simulink model "Batbot_SIM"  (Simulink 7.5)
settings: Solver=ode45  StartTime=0.0  StopTime=5  FixedStep=0.1  RelTol=1e-3
values from neighbouring files (symbols this model uses):
  F_flapping = 1000    [SimulationFB.m]
  step_2 = tf/(col-1)    [SimulationFB.m]    (also in inverse_kinematicsFULLFB.m = 0.0114285714286)
libraries: mblibv1 x76, motdrv_lib x8, simulink x7
(part 3 of 3)

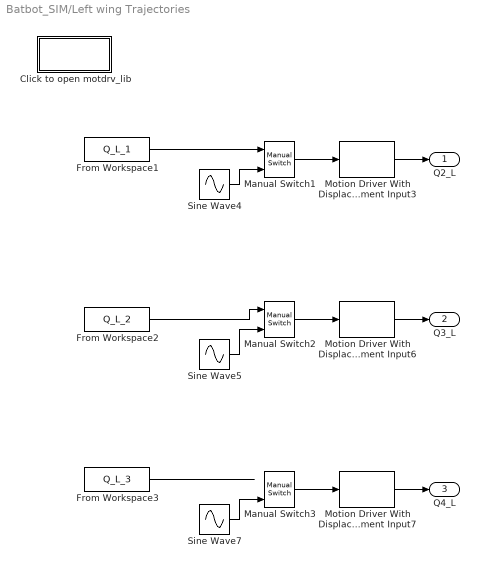
== system Batbot_SIM/Left wing Trajectories  ==
  Click to open motdrv_lib : Subsystem
      settings: OpenFcn=open_system('motdrv_lib');
      mask Type: Double-click to open motdrv_lib
      mask Display: disp('motdrv_lib');
  From Workspace1 : FromWorkspace  VariableName=Q_L_1  SampleTime=step_2  OutputAfterFinalValue=Setting to zero
  From Workspace2 : FromWorkspace  VariableName=Q_L_2  SampleTime=step_2  OutputAfterFinalValue=Setting to zero
  From Workspace3 : FromWorkspace  VariableName=Q_L_3  SampleTime=step_2  OutputAfterFinalValue=Setting to zero
  Manual Switch1 : simulink/Signal Routing/Manual Switch  SystemSampleTime=-1  sw=0  action=0  varsize=off
  Manual Switch2 : simulink/Signal Routing/Manual Switch  SystemSampleTime=-1  sw=0  action=0  varsize=off
  Manual Switch3 : simulink/Signal Routing/Manual Switch  SystemSampleTime=-1  sw=0  action=0  varsize=off
  Motion Driver With Displacement Input3 : motdrv_lib/Motion Driver With Displacement Input  SystemSampleTime=-1  InitialDisplacementSource=Dialog  InitialDisplacement=0  InitialVelocity=0  TimeConstant=1e-3
  Motion Driver With Displacement Input6 : motdrv_lib/Motion Driver With Displacement Input  SystemSampleTime=-1  InitialDisplacementSource=Dialog  InitialDisplacement=0  InitialVelocity=0  TimeConstant=1e-3
  Motion Driver With Displacement Input7 : motdrv_lib/Motion Driver With Displacement Input  SystemSampleTime=-1  InitialDisplacementSource=Dialog  InitialDisplacement=0  InitialVelocity=0  TimeConstant=1e-3
  Sine Wave4 : Sin  Amplitude=40  Bias=0  Frequency=1000  Phase=0  Samples=10  SampleTime=0  Offset=0
  Sine Wave5 : Sin  Amplitude=-60  Bias=0  Frequency=1000  Phase=0  Samples=10  SampleTime=0  Offset=0
  Sine Wave7 : Sin  Amplitude=-60  Bias=0  Frequency=1000  Phase=0  Samples=10  SampleTime=0  Offset=0
  Q2_L : Outport  OutDataType=fixdt(1, 16)  OutScaling=2^0
  Q3_L : Outport  Port=2  OutDataType=fixdt(1, 16)  OutScaling=2^0
  Q4_L : Outport  Port=3  OutDataType=fixdt(1, 16)  OutScaling=2^0
  wires:
  Motion Driver With Displacement Input3/1 -> Q2_L/1
  Motion Driver With Displacement Input6/1 -> Q3_L/1
  Motion Driver With Displacement Input7/1 -> Q4_L/1
  Manual Switch3/1 -> Motion Driver With Displacement Input7/1
  Sine Wave7/1 -> Manual Switch3/2
  Sine Wave5/1 -> Manual Switch2/2
  Sine Wave4/1 -> Manual Switch1/2
  Manual Switch1/1 -> Motion Driver With Displacement Input3/1
  Manual Switch2/1 -> Motion Driver With Displacement Input6/1
  From Workspace1/1 -> Manual Switch1/1
  From Workspace2/1 -> Manual Switch2/1
  From Workspace3/1 -> ?

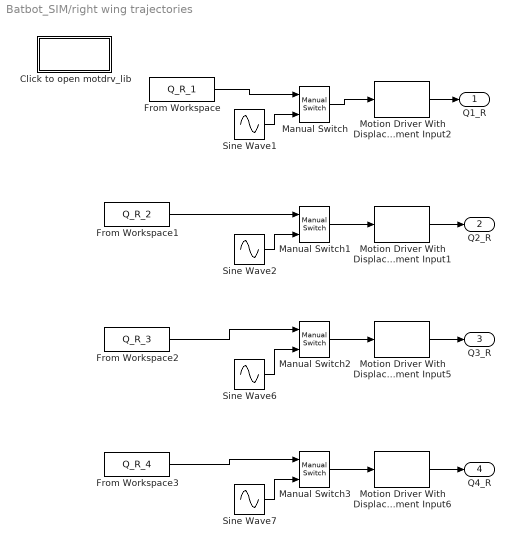
== system Batbot_SIM/right wing trajectories ==
  Click to open motdrv_lib : Subsystem
      settings: OpenFcn=open_system('motdrv_lib');
      mask Type: Double-click to open motdrv_lib
      mask Display: disp('motdrv_lib');
  From Workspace : FromWorkspace  VariableName=Q_R_1  SampleTime=step_2  OutputAfterFinalValue=Setting to zero
  From Workspace1 : FromWorkspace  VariableName=Q_R_2  SampleTime=step_2  OutputAfterFinalValue=Setting to zero
  From Workspace2 : FromWorkspace  VariableName=Q_R_3  SampleTime=step_2  OutputAfterFinalValue=Setting to zero
  From Workspace3 : FromWorkspace  VariableName=Q_R_4  SampleTime=step_2  OutputAfterFinalValue=Setting to zero
  Manual Switch{,1..3} (4 alike) : simulink/Signal Routing/Manual Switch  SystemSampleTime=-1  sw=0  action=0  varsize=off
  Motion Driver With Displacement Input{1..2,5..6} (4 alike) : motdrv_lib/Motion Driver With Displacement Input  SystemSampleTime=-1  InitialDisplacementSource=Dialog  InitialDisplacement=0  InitialVelocity=0  TimeConstant=1e-3
  Sine Wave1 : Sin  Amplitude=200  Bias=0  Frequency=F_flapping  Phase=0  Samples=10  SampleTime=0  Offset=0
  Sine Wave2 : Sin  Amplitude=40  Bias=0  Frequency=1000  Phase=0  Samples=10  SampleTime=0  Offset=0
  Sine Wave6 : Sin  Amplitude=60  Bias=0  Frequency=1000  Phase=0  Samples=10  SampleTime=0  Offset=0
  Sine Wave7 : Sin  Amplitude=60  Bias=0  Frequency=1000  Phase=0  Samples=10  SampleTime=0  Offset=0
  Q1_R : Outport  OutDataType=fixdt(1, 16)  OutScaling=2^0
  Q2_R : Outport  Port=2  OutDataType=fixdt(1, 16)  OutScaling=2^0
  Q3_R : Outport  Port=3  OutDataType=fixdt(1, 16)  OutScaling=2^0
  Q4_R : Outport  Port=4  OutDataType=fixdt(1, 16)  OutScaling=2^0
  wires:
  Motion Driver With Displacement Input1/1 -> Q2_R/1
  Motion Driver With Displacement Input5/1 -> Q3_R/1
  Motion Driver With Displacement Input6/1 -> Q4_R/1
  Motion Driver With Displacement Input2/1 -> Q1_R/1
  Manual Switch3/1 -> Motion Driver With Displacement Input6/1
  Sine Wave7/1 -> Manual Switch3/2
  Sine Wave6/1 -> Manual Switch2/2
  Sine Wave2/1 -> Manual Switch1/2
  Sine Wave1/1 -> Manual Switch/2
  Manual Switch/1 -> Motion Driver With Displacement Input2/1
  Manual Switch1/1 -> Motion Driver With Displacement Input1/1
  Manual Switch2/1 -> Motion Driver With Displacement Input5/1
  From Workspace/1 -> Manual Switch/1
  From Workspace1/1 -> Manual Switch1/1
  From Workspace2/1 -> Manual Switch2/1
  From Workspace3/1 -> Manual Switch3/1

== system Batbot_SIM/Batbot Mechanics + Dynamics/Click to open motdrv_lib ==

== system Batbot_SIM/Left wing Trajectories /Click to open motdrv_lib ==

== system Batbot_SIM/right wing trajectories/Click to open motdrv_lib ==
